simulink library "LumAerospaceBlockset_Animation"  (R2021a)
settings: Solver=ode45  StartTime=0.0  StopTime=10.0  RelTol=1e-3  EnableMultiTasking=on
undefined symbols (not defined in the file or in its folder): payload, SendPositionOrientationAndCameraViewToXPlaneOverUDP, SendPositionOrientationToXPlaneOverUDP, simulation
libraries: aerolibanimutils x3, aerolibutil x2, vrlib x1, LumAerospaceBlockset_Payloads x1
settings Model: Creator=Christopher  LastModifiedBy=chris
settings SolverCC: AlgebraicLoopSolver=TrustRegion
settings DataIOCC: LimitDataPoints=on  SaveFormat=Array  ReturnWorkspaceOutputs=off
settings OptimizationCC: LifeSpan=inf
settings DebuggingCC: SolverPrmCheckMsg=warning  SFUnexpectedBacktrackingDiag=warning  SFNoUnconditionalDefaultTransitionDiag=warning  SFExecutionAtInitializationDiag=none  SFMachineParentedDataDiag=warning  ArithmeticOperatorsInVariantConditions=warning
settings HardwareCC: ProdBitPerPointer=32  ProdBitPerSizeT=32  ProdBitPerPtrDiffT=32  ProdLargestAtomicFloat=None  ProdIntDivRoundTo=Undefined  ProdEndianess=Unspecified  ProdWordSize=32  ProdHWDeviceType=32-bit Generic
settings ModelReferenceCC: PropagateSignalLabelsOutOfModel=off
settings SFSimCC: SimUseLocalCustomCode=off  CustomCodeUndefinedFunction=UseInterfaceOnly
settings RTWCC: RTWUseLocalCustomCode=off
settings CodeAppCC: StateflowObjectComments=on
settings GRTTargetCC: TargetLangStandard=C89/C90 (ANSI)
settings ConfigComp: CovMetricSettings=dw  CovSaveCumulativeToWorkspaceVar=on  CovSaveSingleToWorkspaceVar=on  CovExternalEMLEnable=off  CovSFcnEnable=off

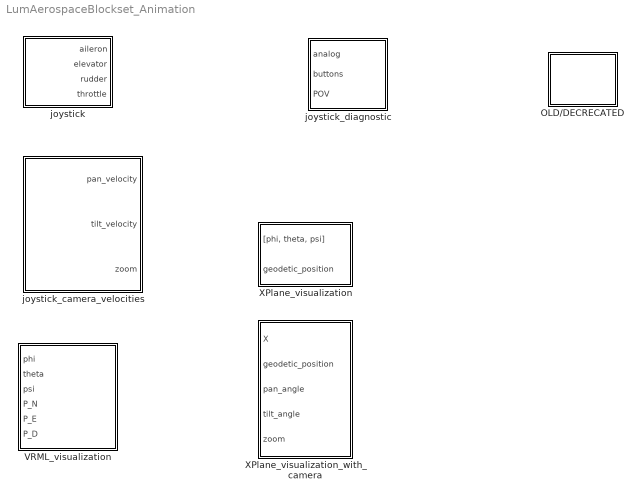
== system LumAerospaceBlockset_Animation ==
  OLD/DECRECATED : Subsystem
  VRML_visualization : Subsystem
      mask help:
      | Visualize the aircraft using a VRML sink.
      |
      | Note: Simulink should open up the VRML sink and it should display the aircraft model in a separate window.  If this does not occur, you may need to look under the mask and through down through subsystems until you find the VR Sink block.  Double click on this block to open the aircraft animation window.
      |
      | Further note that Simulink may close the VRML sink the first time it is run (it may display a warning with verbiage about 'Virtual world has been closed from outside of Simulink.'.  If this occurs, simply repeat the procedure of looking under the mask and double clicking on the VR Sink.
      |
      | Note that this block is derived from the Matlab HL-20 Airframe and Controller demo (type 'aeroblk_HL20' into the command window).
      |
      | INPUTS: -phi: bank angle (rad)
      |         -theta: pitch angle (rad)
      |         -psi: yaw angle (rad)
      |         -P_N:   position north (m)
      |         -P_E:   position down (m)
      |         -P_D:   position down (m)
      |
      | OUTPUTS: -none
  XPlane_visualization : Subsystem  mask{IP_address=simulation.x_plane.state_visualization.IP_address, plugin_listening_port_number=simulation.x_plane.state_visualization.plugin_listening_port_number, numDigitsOfPrecision=simulation.x_plane.state_visualization.numDigitsOfPrecision}
      mask prompts: IP_address "String of X-Plane machine IP address (i.e. '192.168..112')"; plugin_listening_port_number "Port number that the X-Plane plugin is expecting to receive UDP messages on (i.e. 49003)"; numDigitsOfPrecision "Number of degrees of precision to transmit a string representation of a number over UDP (i.e. 10)"
      mask help:
      | Visualize state of aircraft using X-Plane.
      |
      | The machine running X-Plane should have a plugin operating which disables the internal X-Plane physics engine and listens to state information over UDP (which it then applies to the simulator).
      |
      | INPUT:
      | -3-by-1 vector of the euler angles [phi (rad);theta (rad);psi (rad)]
      | -geodetic_position: 3-by-1 vector of [latitude (rad); longitude (rad); altitude (m)]
      |
      | OUTPUT: -none
      |
      | Christopher Lum
      | lum@uw.edu
  XPlane_visualization_with_camera : Subsystem  mask{IP_address=simulation.x_plane.camera_visualization.IP_address, plugin_listening_port_number=simulation.x_plane.camera_visualization.plugin_listening_port_number, numDigitsOfPrecision=simulation.x_plane.camera_visualization.numDigitsOfPrecision}
      mask prompts: IP_address "String of X-Plane machine IP address (i.e. '192.47..102')"; plugin_listening_port_number "Port number that the X-Plane plugin is expecting to receive UDP messages on (i.e. 49004)"; numDigitsOfPrecision "Number of degrees of precision to transmit a string representation of a number over UDP (i.e. 10)"
      mask help:
      | Visualize state of aircraft using X-Plane.
      |
      | This includes support for a camera which is located at the same location as the aircraft.
      |
      | The machine running X-Plane should have a plugin operating which disables the internal X-Plane physics engine and listens to state information over UDP (which it then applies to the simulator).
      |
      | INPUT:  -X:             12-by-1 vector of the state [u (m/s);v (m/s);w (m/s);p (rad/s);q (rad/s);r (rad/s);phi (rad);theta (rad);psi (rad);P_N (m);P_E (m);P_D (m)]
      |         -geodetic_position: 3-by-1 vector of [latitude (rad); longitude (rad); altitude (m)]
      |         -pan_angle:     pan angle of camera (rad)
      |         -tilt_angle:    tilt angle of camera (rad)
      |         -zoom:          zoom factor (1 = no zoom, 2 = double zoom)
      |
      | OUTPUT: -none
      |
      | VALIDATION: -unit test
  joystick : Subsystem  mask{joystickID=Joystick1, max_aileron_deflection=30*pi/180, max_elevator_deflection=20*pi/180, max_rudder_deflection=20*pi/180, sample_time=simulation.sample_time}
      mask prompts: joystickID "Joystick ID"; max_aileron_deflection "max aileron deflection (radians)"; max_elevator_deflection "max elevator deflection (radians)"; max_rudder_deflection "max rudder deflection (rad)"; sample_time "Sample time (sec)"
      mask help:
      | Allows input from the joystick to be mapped to control surface deflections.
      |
      | INPUTS: -none
      |
      | OUTPUTS:    -aileron:   aileron angle (rad)
      |             -elevator:  elevator angle (rad)
      |             -rudder:    rudder angle (rad)
      |             -throttle:  throttle position (in range [0,1])
      mask TypeOptions joystickID: Joystick1 | Joystick2 | None
      mask Callback joystickID: animation_joystickID_CB(gcb)
      mask Display: image('JoystickIcon.png')
  joystick_camera_velocities : Subsystem  mask{joystickID=Joystick1, sample_time=simulation.sample_time, axis_deadzone_percentage=payload.camera.velocity_control_axis_deadzone_percent, max_pan_rate=payload.camera.pan_rate, max_tilt_rate=payload.camera.tilt_rate, max_zoom=payload.camera.zoom_max, min_zoom=payload.camera.zoom_min}
      mask prompts: joystickID "Joystick ID"; sample_time "Sample time (sec)"; axis_deadzone_percentage "Joystick deadzone percentage (in range [0,1])"; max_pan_rate "Maximum pan rate (rad/s)"; max_tilt_rate "Maximum tilt rate (rad/s)"; max_zoom "Maximum zoom (unitless)"; min_zoom "Minimum zoom (unitless)"
      mask help:
      | Outputs the desired camera angle rates and zoom factors for a camera system.
      |
      | Output velocities will be zero until the joystick leaves the specified deadzone.
      | For example, if the deadzone range is 0.05, the joystick must deflect more than 5% of the full range before the outputs will be non-zero.
      |
      | INPUT:  -none
      |
      | OUTPUT: -pan_angle:     desired pan angle (rad)
      |         -tilt_angle:    desired tilt angle (rad)
      |         -zoom:          desired zoom factor (unitless)
      mask TypeOptions joystickID: Joystick1 | Joystick2 | None
      mask Callback joystickID: animation_joystickID_CB(gcb)
      mask DialogControl ParameterTabVar0 Prompt: Joystick
      mask DialogControl ParameterTabVar01 Prompt: Camera
  joystick_diagnostic : Subsystem

== system LumAerospaceBlockset_Animation/OLD//DECRECATED ==
  joystick_diagnostic : Subsystem
  joystick_with_buttons_as_vector : Subsystem
      mask help:
      | Does the same as the 'Pilot Joystick All' block except the buttons are broken out into individual signals instead of a single uint32 word.
      |
      | INPUTS: -none
      |
      | OUTPUTS:    -analog:    same as 'Pilot Joystick All' block
      |             -buttons:   32x1 vector of button states
      |             -POV:       same as 'Pilot Joystick All' block

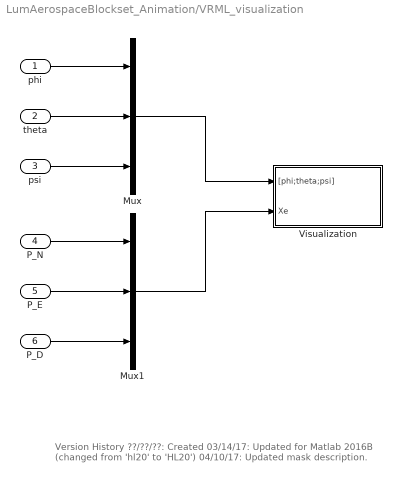
== system LumAerospaceBlockset_Animation/VRML_visualization ==
  note: Version History
      | ??/??/??: Created
      | 03/14/17: Updated for Matlab 2016B (changed from 'hl20' to 'HL20')
      | 04/10/17: Updated mask description.
  phi : Inport
  theta : Inport  Port=2
  psi : Inport  Port=3
  P_N : Inport  Port=4
  P_E : Inport  Port=5
  P_D : Inport  Port=6
  Mux : Mux  Inputs=3
  Mux1 : Mux  Inputs=3
  Visualization : Subsystem
  wires:
  phi/1 -> Mux/1
  theta/1 -> Mux/2
  psi/1 -> Mux/3
  P_N/1 -> Mux1/1
  P_D/1 -> Mux1/3
  P_E/1 -> Mux1/2
  Mux/1 -> Visualization/1("[phi;theta;psi]")
  Mux1/1 -> Visualization/2(Xe)

== system LumAerospaceBlockset_Animation/XPlane_visualization ==
  note: Version History
      | ??/??/??: Created
      | 06/02/20: Changed interface to use only phi, theta, psi.  Updated mask documentation
  "[phi, theta, psi]" : Inport
  geodetic_position : Inport  Port=2
  Demux : Demux  Outputs=3
  Demux5 : Demux  Outputs=3
  MATLAB Fcn : MATLABFcn  MATLABFcn=SendPositionOrientationToXPlaneOverUDP(u, IP_address, plugin_listening_port_number, numDigitsOfPrecision)  OutputDimensions=0
  Mux : Mux  Inputs=6
  wires:
  Mux/1 -> MATLAB Fcn/1
  geodetic_position/1 -> Demux5/1
  "[phi, theta, psi]"/1 -> Demux/1
  Demux/1 -> Mux/1  "phi (rad)"
  Demux/2 -> Mux/2  "theta (rad)"
  Demux/3 -> Mux/3  "psi (rad)"
  Demux5/1 -> Mux/4  "latitude (rad)"
  Demux5/2 -> Mux/5  "longitude (rad)"
  Demux5/3 -> Mux/6  "altitutde (m)"

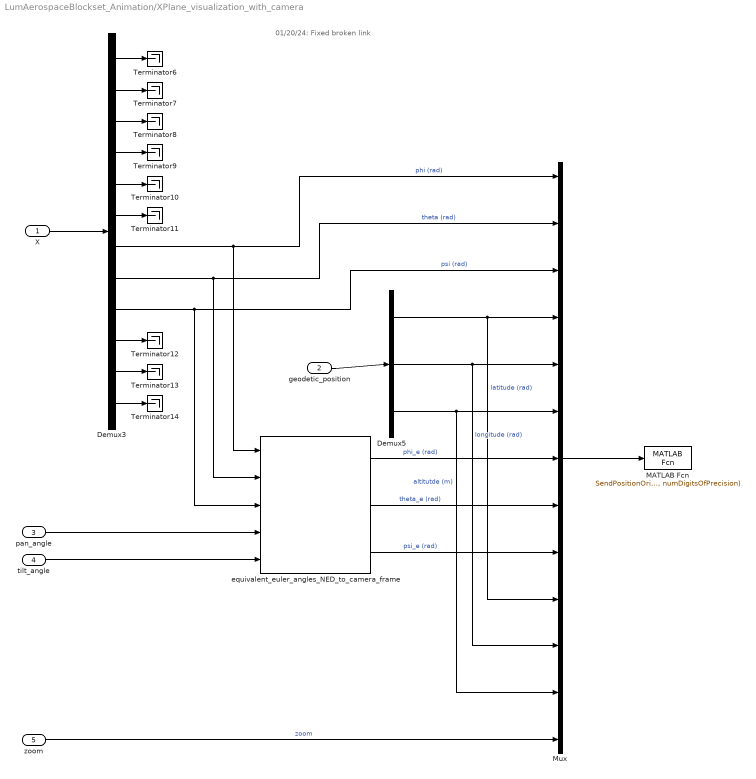
== system LumAerospaceBlockset_Animation/XPlane_visualization_with_camera ==
  note: 01/20/24: Fixed broken link
  X : Inport
  geodetic_position : Inport  Port=2
  pan_angle : Inport  Port=3
  tilt_angle : Inport  Port=4
  zoom : Inport  Port=5
  Demux3 : Demux  Outputs=12
  Demux5 : Demux  Outputs=3
  MATLAB Fcn : MATLABFcn  MATLABFcn=SendPositionOrientationAndCameraViewToXPlaneOverUDP(u, IP_address, plugin_listening_port_number, numDigitsOfPrecision)  OutputDimensions=0
  Mux : Mux  Inputs=13
  Terminator{6..14} (9 alike) : Terminator
  equivalent_euler_angles_NED_to_camera_frame : LumAerospaceBlockset_Payloads/equivalent_euler_angles_NED_to_camera_frame
  wires:
  Mux/1 -> MATLAB Fcn/1
  X/1 -> Demux3/1
  pan_angle/1 -> equivalent_euler_angles_NED_to_camera_frame/4
  tilt_angle/1 -> equivalent_euler_angles_NED_to_camera_frame/5
  equivalent_euler_angles_NED_to_camera_frame/1 -> Mux/7  "phi_e (rad)"
  equivalent_euler_angles_NED_to_camera_frame/2 -> Mux/8  "theta_e (rad)"
  equivalent_euler_angles_NED_to_camera_frame/3 -> Mux/9  "psi_e (rad)"
  zoom/1 -> Mux/13  "zoom"
  Demux5/1 -> Mux/4, Mux/10  "latitude (rad)"
  Demux5/3 -> Mux/6, Mux/12  "altitutde (m)"
  geodetic_position/1 -> Demux5/1
  Demux3/1 -> Terminator6/1
  Demux3/2 -> Terminator7/1
  Demux3/3 -> Terminator8/1
  Demux3/4 -> Terminator9/1
  Demux3/5 -> Terminator10/1
  Demux3/6 -> Terminator11/1
  Demux3/10 -> Terminator12/1
  Demux3/11 -> Terminator13/1
  Demux3/12 -> Terminator14/1
  Demux3/7 -> equivalent_euler_angles_NED_to_camera_frame/1, Mux/1  "phi (rad)"
  Demux3/8 -> equivalent_euler_angles_NED_to_camera_frame/2, Mux/2  "theta (rad)"
  Demux3/9 -> equivalent_euler_angles_NED_to_camera_frame/3, Mux/3  "psi (rad)"
  Demux5/2 -> Mux/5, Mux/11  "longitude (rad)"

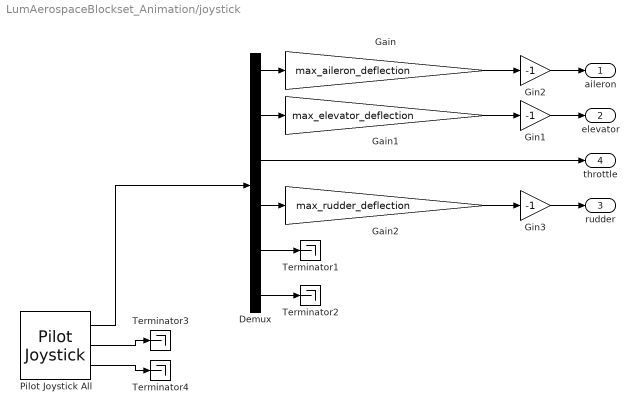
== system LumAerospaceBlockset_Animation/joystick ==
  Demux : Demux  Outputs=6
  Gain : Gain  Gain=max_aileron_deflection
  Gain1 : Gain  Gain=max_elevator_deflection
  Gain2 : Gain  Gain=max_rudder_deflection
  Gin1 : Gain  Gain=-1
  Gin2 : Gain  Gain=-1
  Gin3 : Gain  Gain=-1
  Pilot Joystick All : aerolibanimutils/Pilot Joystick  JoystickID=Joystick1  OutputConfiguration=AllOutputs  SampleTime=sample_time
  Terminator{1..4} (4 alike) : Terminator
  aileron : Outport  VectorParamsAs1DForOutWhenUnconnected=off
  elevator : Outport  Port=2  VectorParamsAs1DForOutWhenUnconnected=off
  rudder : Outport  Port=3  VectorParamsAs1DForOutWhenUnconnected=off
  throttle : Outport  Port=4  VectorParamsAs1DForOutWhenUnconnected=off
  wires:
  Pilot Joystick All/1 -> Demux/1
  Demux/4 -> Gain2/1
  Demux/5 -> Terminator1/1
  Demux/6 -> Terminator2/1
  Demux/1 -> Gain/1
  Demux/2 -> Gain1/1
  Demux/3 -> throttle/1
  Gain/1 -> Gin2/1
  Gain1/1 -> Gin1/1
  Gin2/1 -> aileron/1
  Gin1/1 -> elevator/1
  Pilot Joystick All/2 -> Terminator3/1
  Pilot Joystick All/3 -> Terminator4/1
  Gain2/1 -> Gin3/1
  Gin3/1 -> rudder/1

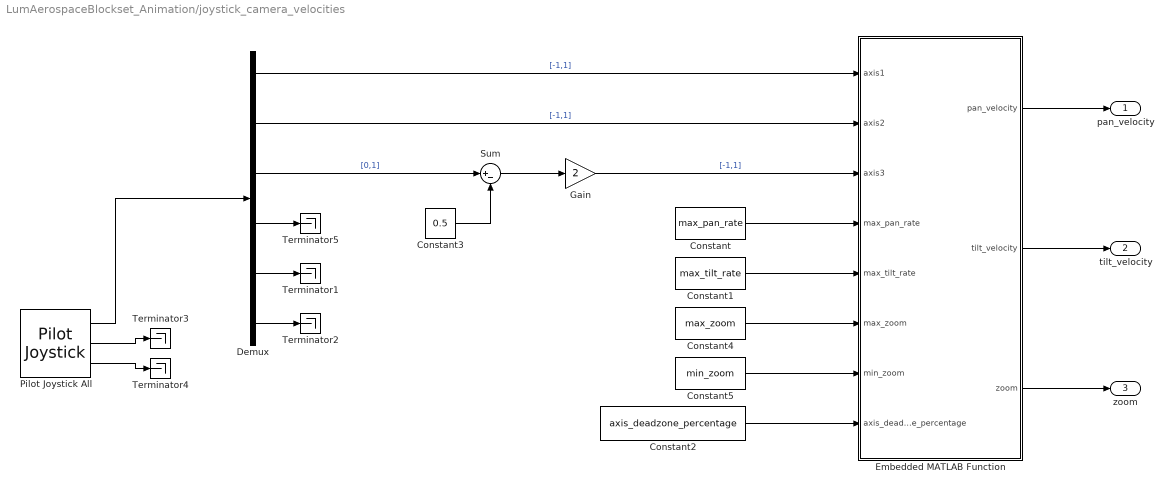
== system LumAerospaceBlockset_Animation/joystick_camera_velocities ==
  Constant : Constant  Value=max_pan_rate
  Constant1 : Constant  Value=max_tilt_rate
  Constant2 : Constant  Value=axis_deadzone_percentage
  Constant3 : Constant  Value=0.5
  Constant4 : Constant  Value=max_zoom
  Constant5 : Constant  Value=min_zoom
  Demux : Demux  Outputs=6
  Embedded MATLAB Function : MATLAB Function  TreatAsAtomicUnit=on
  Gain : Gain  Gain=2
  Pilot Joystick All : aerolibanimutils/Pilot Joystick  JoystickID=Joystick1  OutputConfiguration=AllOutputs  SampleTime=sample_time
  Sum : Sum  Inputs=|+-
  Terminator{1..5} (5 alike) : Terminator
  pan_velocity : Outport  VectorParamsAs1DForOutWhenUnconnected=off
  tilt_velocity : Outport  Port=2  VectorParamsAs1DForOutWhenUnconnected=off
  zoom : Outport  Port=3  VectorParamsAs1DForOutWhenUnconnected=off
  wires:
  Constant2/1 -> Embedded MATLAB Function/8(axis_deadzone_percentage)
  Constant5/1 -> Embedded MATLAB Function/7(min_zoom)
  Constant4/1 -> Embedded MATLAB Function/6(max_zoom)
  Demux/1 -> Embedded MATLAB Function/1(axis1)  "[-1,1]"
  Demux/2 -> Embedded MATLAB Function/2(axis2)  "[-1,1]"
  Demux/3 -> Sum/1  "[0,1]"
  Constant/1 -> Embedded MATLAB Function/4(max_pan_rate)
  Constant1/1 -> Embedded MATLAB Function/5(max_tilt_rate)
  Embedded MATLAB Function/1(pan_velocity) -> pan_velocity/1
  Embedded MATLAB Function/2(tilt_velocity) -> tilt_velocity/1
  Embedded MATLAB Function/3(zoom) -> zoom/1
  Pilot Joystick All/1 -> Demux/1
  Demux/4 -> Terminator5/1
  Demux/5 -> Terminator1/1
  Demux/6 -> Terminator2/1
  Pilot Joystick All/2 -> Terminator3/1
  Pilot Joystick All/3 -> Terminator4/1
  Sum/1 -> Gain/1
  Constant3/1 -> Sum/2
  Gain/1 -> Embedded MATLAB Function/3(axis3)  "[-1,1]"

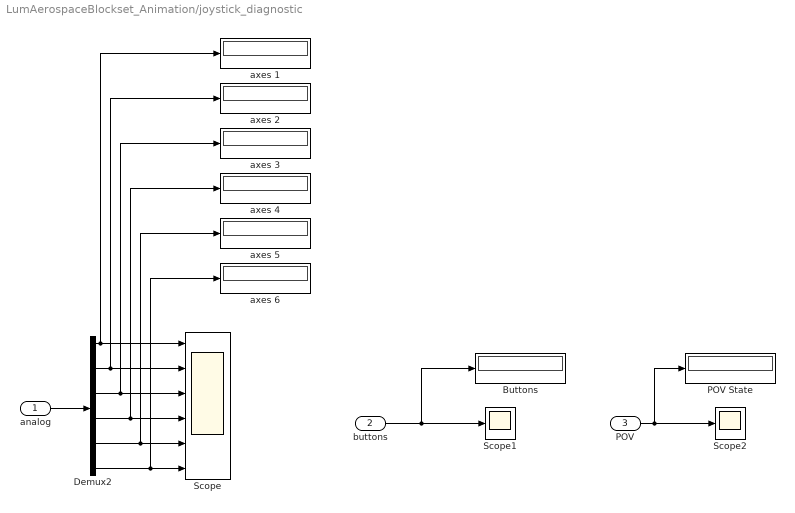
== system LumAerospaceBlockset_Animation/joystick_diagnostic ==
  analog : Inport
  buttons : Inport  Port=2
  POV : Inport  Port=3
  Buttons : Display
  Demux2 : Demux  Outputs=6
      settings: DisplayOption=none
  POV State : Display
  Scope : Scope  NumInputPorts=6
  Scope1 : Scope
  Scope2 : Scope
  axes {1..6} (6 alike) : Display
  wires:
  POV/1 -> Scope2/1, POV State/1
  Demux2/6 -> axes 6/1, Scope/6
  Demux2/5 -> axes 5/1, Scope/5
  Demux2/4 -> axes 4/1, Scope/4
  Demux2/3 -> axes 3/1, Scope/3
  Demux2/2 -> axes 2/1, Scope/2
  Demux2/1 -> axes 1/1, Scope/1
  analog/1 -> Demux2/1
  buttons/1 -> Buttons/1, Scope1/1

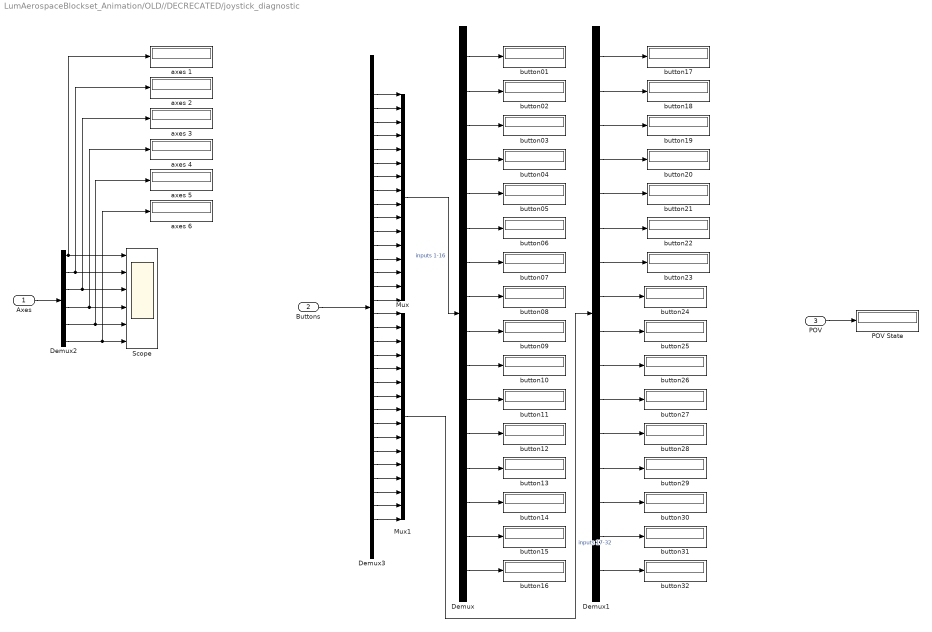
== system LumAerospaceBlockset_Animation/OLD//DECRECATED/joystick_diagnostic ==
  Axes : Inport
  Buttons : Inport  Port=2
  POV : Inport  Port=3
  Demux : Demux  Outputs=16
      settings: DisplayOption=none
  Demux1 : Demux  Outputs=16
      settings: DisplayOption=none
  Demux2 : Demux  Outputs=6
      settings: DisplayOption=none
  Demux3 : Demux  Outputs=32
      settings: DisplayOption=none
  Mux : Mux  Inputs=16
  Mux1 : Mux  Inputs=16
  POV State : Display
  Scope : Scope  NumInputPorts=6
  axes {1..6} (6 alike) : Display
  button01 : Display
  button02 : Display
  button03 : Display
  button04 : Display
  button05 : Display
  button06 : Display
  button07 : Display
  button08 : Display
  button09 : Display
  button{10..32} (23 alike) : Display
  wires:
  POV/1 -> POV State/1
  Demux2/6 -> axes 6/1, Scope/6
  Demux2/5 -> axes 5/1, Scope/5
  Demux2/4 -> axes 4/1, Scope/4
  Demux2/3 -> axes 3/1, Scope/3
  Demux2/2 -> axes 2/1, Scope/2
  Demux2/1 -> axes 1/1, Scope/1
  Axes/1 -> Demux2/1
  Demux1/16 -> button32/1
  Demux1/15 -> button31/1
  Demux1/14 -> button30/1
  Demux1/13 -> button29/1
  Demux1/12 -> button28/1
  Demux1/11 -> button27/1
  Demux1/10 -> button26/1
  Demux1/9 -> button25/1
  Demux1/8 -> button24/1
  Demux1/7 -> button23/1
  Demux1/6 -> button22/1
  Demux1/5 -> button21/1
  Demux1/4 -> button20/1
  Demux1/3 -> button19/1
  Demux1/2 -> button18/1
  Demux1/1 -> button17/1
  Demux/16 -> button16/1
  Demux/15 -> button15/1
  Demux/14 -> button14/1
  Demux/13 -> button13/1
  Demux/12 -> button12/1
  Demux/11 -> button11/1
  Demux/10 -> button10/1
  Demux/9 -> button09/1
  Demux/8 -> button08/1
  Demux/7 -> button07/1
  Demux/6 -> button06/1
  Demux/5 -> button05/1
  Demux/4 -> button04/1
  Demux/3 -> button03/1
  Demux/2 -> button02/1
  Demux/1 -> button01/1
  Mux1/1 -> Demux1/1  "inputs 17-32"
  Demux3/32 -> Mux1/16
  Demux3/31 -> Mux1/15
  Demux3/30 -> Mux1/14
  Demux3/29 -> Mux1/13
  Demux3/28 -> Mux1/12
  Demux3/27 -> Mux1/11
  Demux3/26 -> Mux1/10
  Demux3/25 -> Mux1/9
  Demux3/24 -> Mux1/8
  Demux3/23 -> Mux1/7
  Demux3/22 -> Mux1/6
  Demux3/21 -> Mux1/5
  Demux3/20 -> Mux1/4
  Demux3/19 -> Mux1/3
  Demux3/18 -> Mux1/2
  Demux3/17 -> Mux1/1
  Mux/1 -> Demux/1  "inputs 1-16"
  Demux3/16 -> Mux/16
  Demux3/15 -> Mux/15
  Demux3/14 -> Mux/14
  Demux3/13 -> Mux/13
  Demux3/12 -> Mux/12
  Demux3/11 -> Mux/11
  Demux3/10 -> Mux/10
  Demux3/9 -> Mux/9
  Demux3/8 -> Mux/8
  Demux3/7 -> Mux/7
  Demux3/6 -> Mux/6
  Demux3/5 -> Mux/5
  Demux3/4 -> Mux/4
  Demux3/3 -> Mux/3
  Demux3/2 -> Mux/2
  Demux3/1 -> Mux/1
  Buttons/1 -> Demux3/1

== system LumAerospaceBlockset_Animation/OLD//DECRECATED/joystick_with_buttons_as_vector ==
  Pilot Joystick All : aerolibanimutils/Pilot Joystick  JoystickID=Joystick1  OutputConfiguration=AllOutputs  SampleTime=1/30
  Subsystem : Subsystem
  analog : Outport  VectorParamsAs1DForOutWhenUnconnected=off
  buttons : Outport  Port=2  VectorParamsAs1DForOutWhenUnconnected=off
  POV : Outport  Port=3  VectorParamsAs1DForOutWhenUnconnected=off
  wires:
  Pilot Joystick All/2 -> Subsystem/1(buttons (uint32))
  Pilot Joystick All/1 -> analog/1
  Subsystem/1(buttons (vector)) -> buttons/1
  Pilot Joystick All/3 -> POV/1

== system LumAerospaceBlockset_Animation/VRML_visualization/Visualization ==
  "[phi;theta;psi]" : Inport
  Xe : Inport  Port=2
  Axes to VR Axes : Subsystem
  Euler to VR : Subsystem
  "VR Sink " : vrlib/VR Sink  InstantiateOnLoad=on  SampleTime=-1  ViewEnable=on  RemoteChange=off  RemoteView=off  FieldsWritten=HL20.rotation.4.1.1.double#HL20.translation.3.1.1.double  WorldFileName=aeroblk_HL20.wrl  WorldDescription=aeroblk_HL20  AutoView=on  VideoDimensions=[]  AllowVariableSize=off
  wires:
  "[phi;theta;psi]"/1 -> Euler to VR/1(Euler Angles)
  Xe/1 -> Axes to VR Axes/1(Xe)
  Euler to VR/1(Axis Angle) -> "VR Sink "/1
  Axes to VR Axes/1(Xe VR) -> "VR Sink "/2

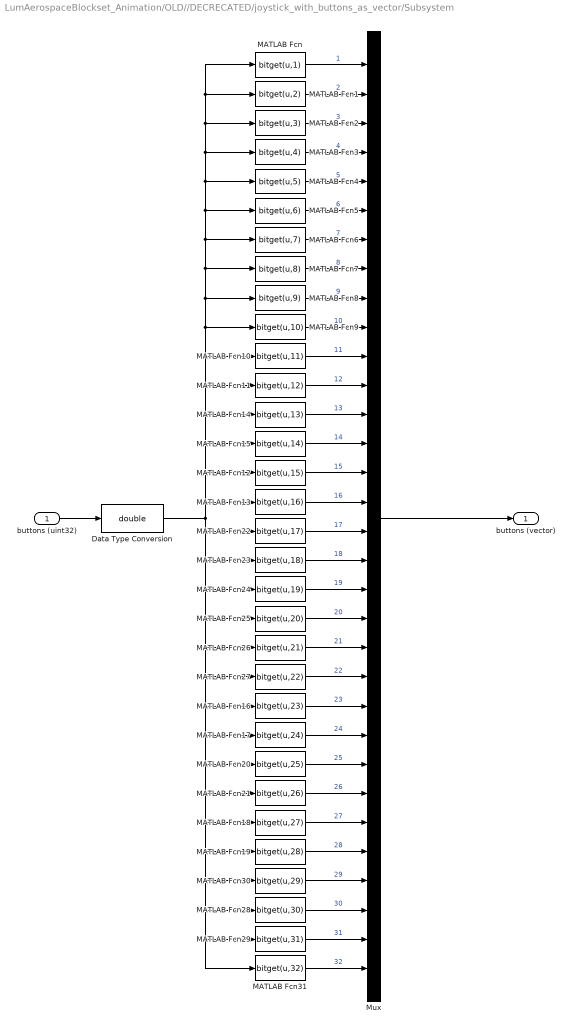
== system LumAerospaceBlockset_Animation/OLD//DECRECATED/joystick_with_buttons_as_vector/Subsystem ==
  buttons (uint32) : Inport
  Data Type Conversion : DataTypeConversion  OutDataTypeStr=double
  MATLAB Fcn : MATLABFcn  MATLABFcn=bitget(u,1)
  MATLAB Fcn1 : MATLABFcn  MATLABFcn=bitget(u,2)
  MATLAB Fcn10 : MATLABFcn  MATLABFcn=bitget(u,11)
  MATLAB Fcn11 : MATLABFcn  MATLABFcn=bitget(u,12)
  MATLAB Fcn12 : MATLABFcn  MATLABFcn=bitget(u,15)
  MATLAB Fcn13 : MATLABFcn  MATLABFcn=bitget(u,16)
  MATLAB Fcn14 : MATLABFcn  MATLABFcn=bitget(u,13)
  MATLAB Fcn15 : MATLABFcn  MATLABFcn=bitget(u,14)
  MATLAB Fcn16 : MATLABFcn  MATLABFcn=bitget(u,23)
  MATLAB Fcn17 : MATLABFcn  MATLABFcn=bitget(u,24)
  MATLAB Fcn18 : MATLABFcn  MATLABFcn=bitget(u,27)
  MATLAB Fcn19 : MATLABFcn  MATLABFcn=bitget(u,28)
  MATLAB Fcn2 : MATLABFcn  MATLABFcn=bitget(u,3)
  MATLAB Fcn20 : MATLABFcn  MATLABFcn=bitget(u,25)
  MATLAB Fcn21 : MATLABFcn  MATLABFcn=bitget(u,26)
  MATLAB Fcn22 : MATLABFcn  MATLABFcn=bitget(u,17)
  MATLAB Fcn23 : MATLABFcn  MATLABFcn=bitget(u,18)
  MATLAB Fcn24 : MATLABFcn  MATLABFcn=bitget(u,19)
  MATLAB Fcn25 : MATLABFcn  MATLABFcn=bitget(u,20)
  MATLAB Fcn26 : MATLABFcn  MATLABFcn=bitget(u,21)
  MATLAB Fcn27 : MATLABFcn  MATLABFcn=bitget(u,22)
  MATLAB Fcn28 : MATLABFcn  MATLABFcn=bitget(u,30)
  MATLAB Fcn29 : MATLABFcn  MATLABFcn=bitget(u,31)
  MATLAB Fcn3 : MATLABFcn  MATLABFcn=bitget(u,4)
  MATLAB Fcn30 : MATLABFcn  MATLABFcn=bitget(u,29)
  MATLAB Fcn31 : MATLABFcn  MATLABFcn=bitget(u,32)
  MATLAB Fcn4 : MATLABFcn  MATLABFcn=bitget(u,5)
  MATLAB Fcn5 : MATLABFcn  MATLABFcn=bitget(u,6)
  MATLAB Fcn6 : MATLABFcn  MATLABFcn=bitget(u,7)
  MATLAB Fcn7 : MATLABFcn  MATLABFcn=bitget(u,8)
  MATLAB Fcn8 : MATLABFcn  MATLABFcn=bitget(u,9)
  MATLAB Fcn9 : MATLABFcn  MATLABFcn=bitget(u,10)
  Mux : Mux  Inputs=32
  buttons (vector) : Outport  VectorParamsAs1DForOutWhenUnconnected=off
  wires:
  buttons (uint32)/1 -> Data Type Conversion/1
  Mux/1 -> buttons (vector)/1
  MATLAB Fcn/1 -> Mux/1  "1"
  MATLAB Fcn1/1 -> Mux/2  "2"
  MATLAB Fcn4/1 -> Mux/5  "5"
  MATLAB Fcn5/1 -> Mux/6  "6"
  MATLAB Fcn2/1 -> Mux/3  "3"
  MATLAB Fcn3/1 -> Mux/4  "4"
  MATLAB Fcn6/1 -> Mux/7  "7"
  MATLAB Fcn7/1 -> Mux/8  "8"
  MATLAB Fcn8/1 -> Mux/9  "9"
  MATLAB Fcn9/1 -> Mux/10  "10"
  MATLAB Fcn10/1 -> Mux/11  "11"
  MATLAB Fcn11/1 -> Mux/12  "12"
  MATLAB Fcn14/1 -> Mux/13  "13"
  MATLAB Fcn15/1 -> Mux/14  "14"
  MATLAB Fcn12/1 -> Mux/15  "15"
  MATLAB Fcn13/1 -> Mux/16  "16"
  MATLAB Fcn22/1 -> Mux/17  "17"
  MATLAB Fcn23/1 -> Mux/18  "18"
  MATLAB Fcn24/1 -> Mux/19  "19"
  MATLAB Fcn25/1 -> Mux/20  "20"
  MATLAB Fcn26/1 -> Mux/21  "21"
  MATLAB Fcn27/1 -> Mux/22  "22"
  MATLAB Fcn16/1 -> Mux/23  "23"
  MATLAB Fcn17/1 -> Mux/24  "24"
  MATLAB Fcn20/1 -> Mux/25  "25"
  MATLAB Fcn21/1 -> Mux/26  "26"
  MATLAB Fcn18/1 -> Mux/27  "27"
  MATLAB Fcn19/1 -> Mux/28  "28"
  MATLAB Fcn30/1 -> Mux/29  "29"
  MATLAB Fcn28/1 -> Mux/30  "30"
  MATLAB Fcn29/1 -> Mux/31  "31"
  MATLAB Fcn31/1 -> Mux/32  "32"
  Data Type Conversion/1 -> MATLAB Fcn30/1, MATLAB Fcn31/1, MATLAB Fcn29/1, MATLAB Fcn28/1, MATLAB Fcn19/1, MATLAB Fcn18/1, MATLAB Fcn21/1, MATLAB Fcn20/1, MATLAB Fcn17/1, MATLAB Fcn16/1, MATLAB Fcn27/1, MATLAB Fcn26/1, MATLAB Fcn25/1, MATLAB Fcn24/1, MATLAB Fcn23/1, MATLAB Fcn22/1, MATLAB Fcn13/1, MATLAB Fcn12/1, MATLAB Fcn15/1, MATLAB Fcn14/1, MATLAB Fcn11/1, MATLAB Fcn10/1, MATLAB Fcn9/1, MATLAB Fcn8/1, MATLAB Fcn7/1, MATLAB Fcn6/1, MATLAB Fcn5/1, MATLAB Fcn4/1, MATLAB Fcn3/1, MATLAB Fcn2/1, MATLAB Fcn/1, MATLAB Fcn1/1

== system LumAerospaceBlockset_Animation/VRML_visualization/Visualization/Axes to VR Axes ==
  Xe : Inport
  Concatenate : Concatenate  NumInputs=3
  Demux : Demux  Outputs=3
      settings: DisplayOption=none
  rad-->deg : Gain  Gain=-1  SaturateOnIntegerOverflow=on  OutDataTypeStr=Inherit: Same as input  ParamDataTypeStr=Inherit: Same as input
  rad-->deg1 : Gain  Gain=-1  SaturateOnIntegerOverflow=on  OutDataTypeStr=Inherit: Same as input  ParamDataTypeStr=Inherit: Same as input
  Xe VR : Outport  VectorParamsAs1DForOutWhenUnconnected=off
  wires:
  Xe/1 -> Demux/1
  Demux/1 -> Concatenate/1
  Demux/2 -> rad-->deg/1
  Demux/3 -> rad-->deg1/1
  Concatenate/1 -> Xe VR/1
  rad-->deg1/1 -> Concatenate/2
  rad-->deg/1 -> Concatenate/3

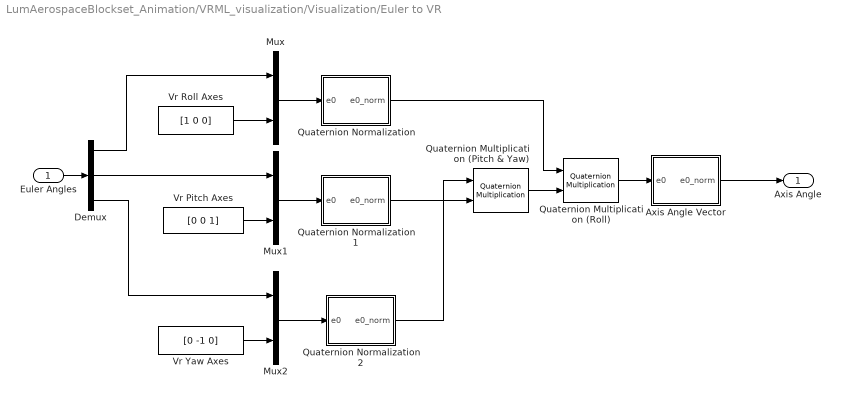
== system LumAerospaceBlockset_Animation/VRML_visualization/Visualization/Euler to VR ==
  Euler Angles : Inport
  Axis Angle Vector : Subsystem
  Demux : Demux  Outputs=3
      settings: DisplayOption=none
  Mux : Mux  Inputs=2
  Mux1 : Mux  Inputs=2
  Mux2 : Mux  Inputs=2
  Quaternion Multiplication (Pitch & Yaw) : aerolibutil/Quaternion Multiplication
  Quaternion Multiplication (Roll) : aerolibutil/Quaternion Multiplication
  Quaternion Normalization : Subsystem
  Quaternion Normalization1 : Subsystem
  Quaternion Normalization2 : Subsystem
  Vr Pitch Axes : Constant  Value=[0 0 1]
  Vr Roll Axes : Constant  Value=[1 0 0]
  Vr Yaw Axes : Constant  Value=[0 -1 0]
  Axis Angle : Outport  VectorParamsAs1DForOutWhenUnconnected=off
  wires:
  Quaternion Multiplication (Roll)/1 -> Axis Angle Vector/1(e0)
  Quaternion Multiplication (Pitch & Yaw)/1 -> Quaternion Multiplication (Roll)/2
  Axis Angle Vector/1(e0_norm) -> Axis Angle/1
  Quaternion Normalization/1(e0_norm) -> Quaternion Multiplication (Roll)/1
  Quaternion Normalization2/1(e0_norm) -> Quaternion Multiplication (Pitch & Yaw)/1
  Quaternion Normalization1/1(e0_norm) -> Quaternion Multiplication (Pitch & Yaw)/2
  Mux2/1 -> Quaternion Normalization2/1(e0)
  Mux1/1 -> Quaternion Normalization1/1(e0)
  Mux/1 -> Quaternion Normalization/1(e0)
  Vr Yaw Axes/1 -> Mux2/2
  Vr Pitch Axes/1 -> Mux1/2
  Vr Roll Axes/1 -> Mux/2
  Euler Angles/1 -> Demux/1
  Demux/1 -> Mux/1
  Demux/2 -> Mux1/1
  Demux/3 -> Mux2/1

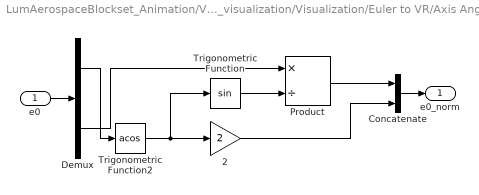
== system LumAerospaceBlockset_Animation/VRML_visualization/Visualization/Euler to VR/Axis Angle Vector ==
  e0 : Inport
  2 : Gain  Gain=2  SaturateOnIntegerOverflow=on  OutDataTypeStr=Inherit: Same as input  ParamDataTypeStr=Inherit: Same as input
  Concatenate : Concatenate
  Demux : Demux  Outputs=[1 3 ]
      settings: DisplayOption=none
  Product : Product  Inputs=*/  InputSameDT=on  SaturateOnIntegerOverflow=on  OutDataTypeStr=Inherit: Same as first input
  Trigonometric Function : Trigonometry
  Trigonometric Function2 : Trigonometry  Operator=acos
  e0_norm : Outport  VectorParamsAs1DForOutWhenUnconnected=off
  wires:
  Demux/1 -> Trigonometric Function2/1
  Demux/2 -> Product/1
  Concatenate/1 -> e0_norm/1
  Product/1 -> Concatenate/1
  2/1 -> Concatenate/2
  Trigonometric Function/1 -> Product/2
  Trigonometric Function2/1 -> Trigonometric Function/1, 2/1
  e0/1 -> Demux/1

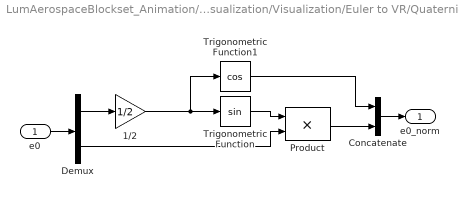
== system LumAerospaceBlockset_Animation/VRML_visualization/Visualization/Euler to VR/Quaternion Normalization ==
  e0 : Inport
  1/2 : Gain  Gain=1/2  SaturateOnIntegerOverflow=on  OutDataTypeStr=Inherit: Same as input  ParamDataTypeStr=Inherit: Same as input
  Concatenate : Concatenate
  Demux : Demux  Outputs=[1 3]
      settings: DisplayOption=none
  Product : Product  InputSameDT=on  SaturateOnIntegerOverflow=on  OutDataTypeStr=Inherit: Same as first input
  Trigonometric Function : Trigonometry
  Trigonometric Function1 : Trigonometry  Operator=cos
  e0_norm : Outport  VectorParamsAs1DForOutWhenUnconnected=off
  wires:
  Trigonometric Function1/1 -> Concatenate/1
  Demux/2 -> Product/2
  Demux/1 -> 1/2/1
  Concatenate/1 -> e0_norm/1
  Product/1 -> Concatenate/2
  Trigonometric Function/1 -> Product/1
  1/2/1 -> Trigonometric Function1/1, Trigonometric Function/1
  e0/1 -> Demux/1

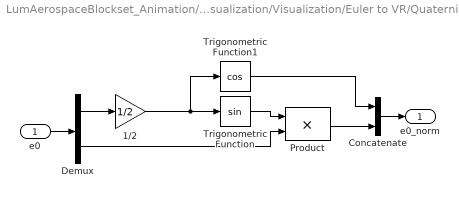
== system LumAerospaceBlockset_Animation/VRML_visualization/Visualization/Euler to VR/Quaternion Normalization1 ==
  e0 : Inport
  1/2 : Gain  Gain=1/2  SaturateOnIntegerOverflow=on  OutDataTypeStr=Inherit: Same as input  ParamDataTypeStr=Inherit: Same as input
  Concatenate : Concatenate
  Demux : Demux  Outputs=[1 3]
      settings: DisplayOption=none
  Product : Product  InputSameDT=on  SaturateOnIntegerOverflow=on  OutDataTypeStr=Inherit: Same as first input
  Trigonometric Function : Trigonometry
  Trigonometric Function1 : Trigonometry  Operator=cos
  e0_norm : Outport  VectorParamsAs1DForOutWhenUnconnected=off
  wires:
  e0/1 -> Demux/1
  1/2/1 -> Trigonometric Function/1, Trigonometric Function1/1
  Trigonometric Function/1 -> Product/1
  Product/1 -> Concatenate/2
  Concatenate/1 -> e0_norm/1
  Demux/1 -> 1/2/1
  Demux/2 -> Product/2
  Trigonometric Function1/1 -> Concatenate/1

== system LumAerospaceBlockset_Animation/VRML_visualization/Visualization/Euler to VR/Quaternion Normalization2 ==
  e0 : Inport
  1/2 : Gain  Gain=1/2  SaturateOnIntegerOverflow=on  OutDataTypeStr=Inherit: Same as input  ParamDataTypeStr=Inherit: Same as input
  Concatenate : Concatenate
  Demux : Demux  Outputs=[1 3]
      settings: DisplayOption=none
  Product : Product  InputSameDT=on  SaturateOnIntegerOverflow=on  OutDataTypeStr=Inherit: Same as first input
  Trigonometric Function : Trigonometry
  Trigonometric Function1 : Trigonometry  Operator=cos
  e0_norm : Outport  VectorParamsAs1DForOutWhenUnconnected=off
  wires:
  Trigonometric Function1/1 -> Concatenate/1
  Demux/2 -> Product/2
  Demux/1 -> 1/2/1
  Concatenate/1 -> e0_norm/1
  Product/1 -> Concatenate/2
  Trigonometric Function/1 -> Product/1
  1/2/1 -> Trigonometric Function1/1, Trigonometric Function/1
  e0/1 -> Demux/1

== matlab function LumAerospaceBlockset_Animation/joystick_camera_velocities/Embedded MATLAB Function ==
  data: axis1 input; pan_velocity output; axis2 input; axis3 input; max_pan_rate input; max_tilt_rate input; max_zoom input; min_zoom input; tilt_velocity output; zoom output; axis_deadzone_percentage input
function [pan_velocity, tilt_velocity, zoom] = fcn(axis1, axis2, axis3, max_pan_rate, max_tilt_rate, max_zoom, min_zoom, axis_deadzone_percentage)
%#eml

%Pan (axis 1)
if(abs(axis1) < axis_deadzone_percentage)
    pan_velocity = 0;
else
    pan_velocity = max_pan_rate*axis1;
end

%Tilt (axis 2)
if(abs(axis2) < axis_deadzone_percentage)
    tilt_velocity = 0;
else
    tilt_velocity  = max_tilt_rate*axis2;
end

%Zoom (axis 3)
slope_zoom = (max_zoom - min_zoom)/(2);
y_intercept_zoom = max_zoom - slope_zoom*1;
zoom = slope_zoom*axis3 + y_intercept_zoom;
